simulink model "VehicleECU"  (R2018b)
settings: configuration reference "Active" (kept outside this file)
undefined symbols (not defined in the file): TUMHealthStatus, TUMStrategyState
settings Model: DataDictionary=VehicleECU.sldd  sg_rtwmakecfg_data=_sglibc_  ExplicitPartitioning=on  Creator=wischnewski  LastModifiedBy=ge34qer

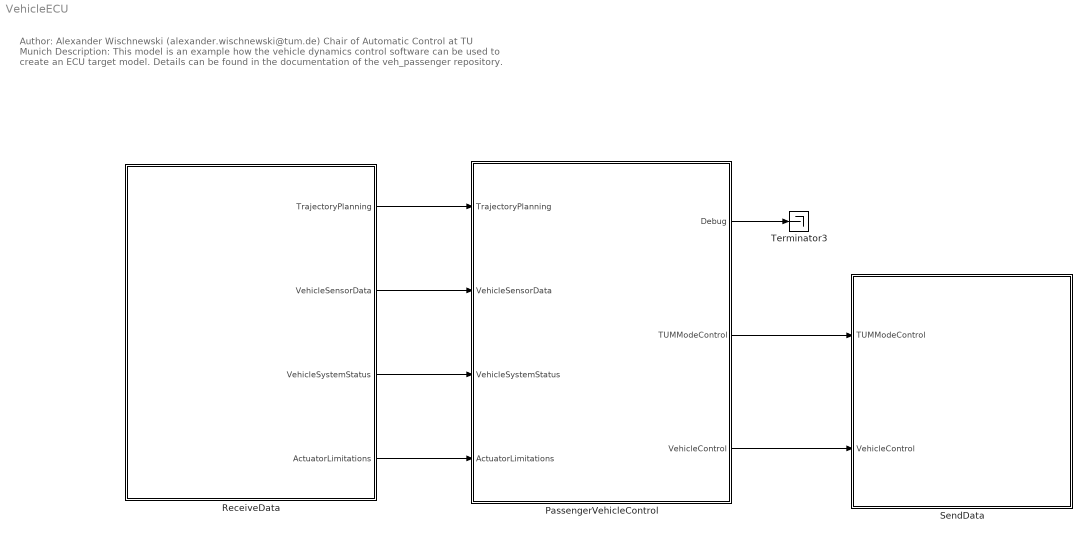
== system VehicleECU ==
  note: Author: Alexander Wischnewski (alexander.wischnewski@tum.de)
      | Chair of Automatic Control at TU Munich
      |
      | Description: This model is an example how the vehicle dynamics control software can be used to create an ECU target model. Details
      | can be found in the documentation of the veh_passenger repository.
  PassengerVehicleControl : Subsystem
  ReceiveData : Subsystem
  SendData : Subsystem
  Terminator3 : Terminator
  wires:
  ReceiveData/1(TrajectoryPlanning) -> PassengerVehicleControl/1(TrajectoryPlanning)
  ReceiveData/2(VehicleSensorData) -> PassengerVehicleControl/2(VehicleSensorData)
  ReceiveData/3(VehicleSystemStatus) -> PassengerVehicleControl/3(VehicleSystemStatus)
  ReceiveData/4(ActuatorLimitations) -> PassengerVehicleControl/4(ActuatorLimitations)
  PassengerVehicleControl/3(VehicleControl) -> SendData/2(VehicleControl)
  PassengerVehicleControl/2(TUMModeControl) -> SendData/1(TUMModeControl)
  PassengerVehicleControl/1(Debug) -> Terminator3/1

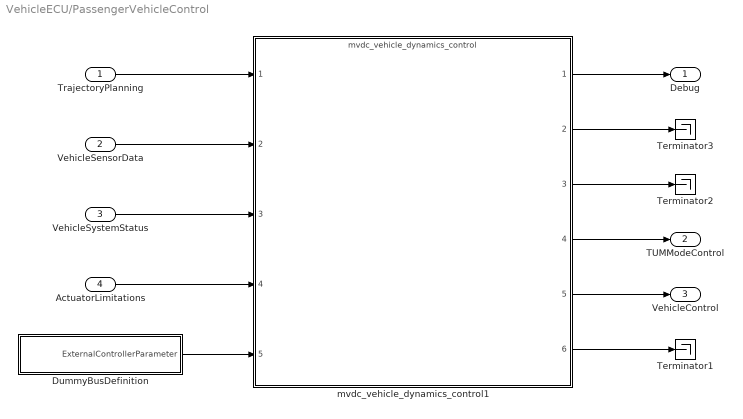
== system VehicleECU/PassengerVehicleControl ==
  TrajectoryPlanning : Inport
  VehicleSensorData : Inport  Port=2
  VehicleSystemStatus : Inport  Port=3
  ActuatorLimitations : Inport  Port=4
  DummyBusDefinition : Subsystem
  Terminator1 : Terminator
  Terminator2 : Terminator
  Terminator3 : Terminator
  mvdc_vehicle_dynamics_control1 : ModelReference  ModelNameDialog=mvdc_vehicle_dynamics_control  SimulationMode=Normal  ModelReferenceVersion=1.726
  Debug : Outport
  TUMModeControl : Outport  Port=2
  VehicleControl : Outport  Port=3
  wires:
  VehicleSystemStatus/1 -> mvdc_vehicle_dynamics_control1/3
  ActuatorLimitations/1 -> mvdc_vehicle_dynamics_control1/4
  VehicleSensorData/1 -> mvdc_vehicle_dynamics_control1/2
  TrajectoryPlanning/1 -> mvdc_vehicle_dynamics_control1/1
  mvdc_vehicle_dynamics_control1/6 -> Terminator1/1
  mvdc_vehicle_dynamics_control1/3 -> Terminator2/1
  mvdc_vehicle_dynamics_control1/2 -> Terminator3/1
  mvdc_vehicle_dynamics_control1/5 -> VehicleControl/1
  mvdc_vehicle_dynamics_control1/4 -> TUMModeControl/1
  DummyBusDefinition/1(ExternalControllerParameter) -> mvdc_vehicle_dynamics_control1/5
  mvdc_vehicle_dynamics_control1/1 -> Debug/1

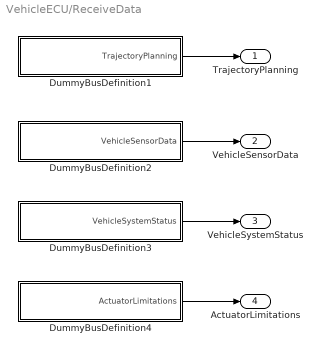
== system VehicleECU/ReceiveData ==
  DummyBusDefinition1 : Subsystem
  DummyBusDefinition2 : Subsystem
  DummyBusDefinition3 : Subsystem
  DummyBusDefinition4 : Subsystem
  TrajectoryPlanning : Outport
  VehicleSensorData : Outport  Port=2
  VehicleSystemStatus : Outport  Port=3
  ActuatorLimitations : Outport  Port=4
  wires:
  DummyBusDefinition4/1(ActuatorLimitations) -> ActuatorLimitations/1
  DummyBusDefinition3/1(VehicleSystemStatus) -> VehicleSystemStatus/1
  DummyBusDefinition2/1(VehicleSensorData) -> VehicleSensorData/1
  DummyBusDefinition1/1(TrajectoryPlanning) -> TrajectoryPlanning/1

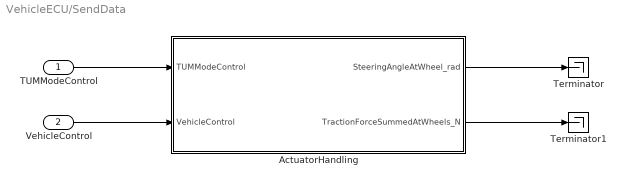
== system VehicleECU/SendData ==
  TUMModeControl : Inport  OutDataTypeStr=Bus: TUMModeControl
  VehicleControl : Inport  Port=2  OutDataTypeStr=Bus: VehicleControl
  ActuatorHandling : Subsystem
  Terminator : Terminator
  Terminator1 : Terminator
  wires:
  TUMModeControl/1 -> ActuatorHandling/1(TUMModeControl)
  VehicleControl/1 -> ActuatorHandling/2(VehicleControl)
  ActuatorHandling/1(SteeringAngleAtWheel_rad) -> Terminator/1
  ActuatorHandling/2(TractionForceSummedAtWheels_N) -> Terminator1/1

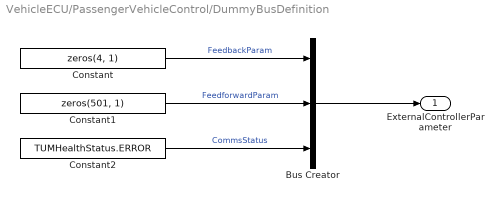
== system VehicleECU/PassengerVehicleControl/DummyBusDefinition ==
  Bus Creator : BusCreator  Inputs=3
  Constant : Constant  Value=zeros(4, 1)
  Constant1 : Constant  Value=zeros(501, 1)
  Constant2 : Constant  Value=TUMHealthStatus.ERROR
  ExternalControllerParameter : Outport
  wires:
  Bus Creator/1 -> ExternalControllerParameter/1
  Constant/1 -> Bus Creator/1  "FeedbackParam"
  Constant1/1 -> Bus Creator/2  "FeedforwardParam"
  Constant2/1 -> Bus Creator/3  "CommsStatus"

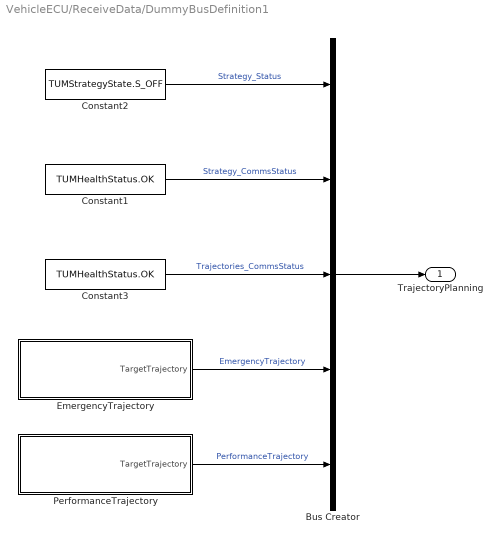
== system VehicleECU/ReceiveData/DummyBusDefinition1 ==
  Bus Creator : BusCreator  Inputs=5  OutDataTypeStr=Bus: TrajectoryPlanning
      settings: InheritFromInputs=off
  Constant1 : Constant  Value=TUMHealthStatus.OK
  Constant2 : Constant  Value=TUMStrategyState.S_OFF
  Constant3 : Constant  Value=TUMHealthStatus.OK
  EmergencyTrajectory : Subsystem  Priority=1000
  PerformanceTrajectory : Subsystem  Priority=1000
  TrajectoryPlanning : Outport
  wires:
  EmergencyTrajectory/1(TargetTrajectory) -> Bus Creator/4  "EmergencyTrajectory"
  Constant2/1 -> Bus Creator/1  "Strategy_Status"
  Constant1/1 -> Bus Creator/2  "Strategy_CommsStatus"
  Bus Creator/1 -> TrajectoryPlanning/1
  Constant3/1 -> Bus Creator/3  "Trajectories_CommsStatus"
  PerformanceTrajectory/1(TargetTrajectory) -> Bus Creator/5  "PerformanceTrajectory"

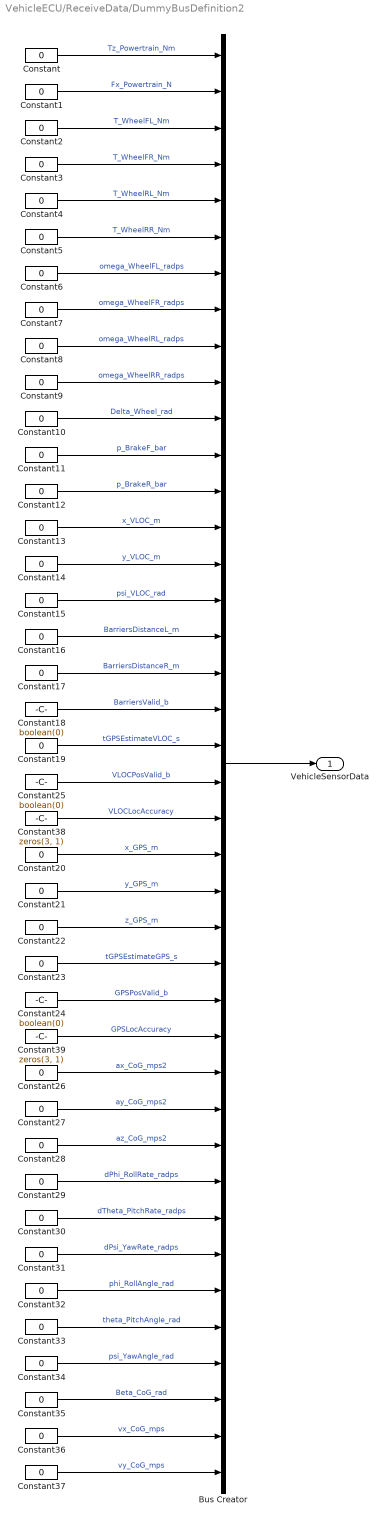
== system VehicleECU/ReceiveData/DummyBusDefinition2 ==
  Bus Creator : BusCreator  Inputs=40
  Constant{,1..17,19..23,26..37} (35 alike) : Constant  Value=0
  Constant18 : Constant  Value=boolean(0)
  Constant24 : Constant  Value=boolean(0)
  Constant25 : Constant  Value=boolean(0)
  Constant38 : Constant  Value=zeros(3, 1)
  Constant39 : Constant  Value=zeros(3, 1)
  VehicleSensorData : Outport
  wires:
  Bus Creator/1 -> VehicleSensorData/1
  Constant/1 -> Bus Creator/1  "Tz_Powertrain_Nm"
  Constant1/1 -> Bus Creator/2  "Fx_Powertrain_N"
  Constant2/1 -> Bus Creator/3  "T_WheelFL_Nm"
  Constant3/1 -> Bus Creator/4  "T_WheelFR_Nm"
  Constant4/1 -> Bus Creator/5  "T_WheelRL_Nm"
  Constant5/1 -> Bus Creator/6  "T_WheelRR_Nm"
  Constant6/1 -> Bus Creator/7  "omega_WheelFL_radps"
  Constant7/1 -> Bus Creator/8  "omega_WheelFR_radps"
  Constant8/1 -> Bus Creator/9  "omega_WheelRL_radps"
  Constant9/1 -> Bus Creator/10  "omega_WheelRR_radps"
  Constant10/1 -> Bus Creator/11  "Delta_Wheel_rad"
  Constant11/1 -> Bus Creator/12  "p_BrakeF_bar"
  Constant12/1 -> Bus Creator/13  "p_BrakeR_bar"
  Constant13/1 -> Bus Creator/14  "x_VLOC_m"
  Constant14/1 -> Bus Creator/15  "y_VLOC_m"
  Constant15/1 -> Bus Creator/16  "psi_VLOC_rad"
  Constant16/1 -> Bus Creator/17  "BarriersDistanceL_m"
  Constant17/1 -> Bus Creator/18  "BarriersDistanceR_m"
  Constant18/1 -> Bus Creator/19  "BarriersValid_b"
  Constant19/1 -> Bus Creator/20  "tGPSEstimateVLOC_s"
  Constant20/1 -> Bus Creator/23  "x_GPS_m"
  Constant21/1 -> Bus Creator/24  "y_GPS_m"
  Constant22/1 -> Bus Creator/25  "z_GPS_m"
  Constant23/1 -> Bus Creator/26  "tGPSEstimateGPS_s"
  Constant24/1 -> Bus Creator/27  "GPSPosValid_b"
  Constant25/1 -> Bus Creator/21  "VLOCPosValid_b"
  Constant26/1 -> Bus Creator/29  "ax_CoG_mps2"
  Constant27/1 -> Bus Creator/30  "ay_CoG_mps2"
  Constant28/1 -> Bus Creator/31  "az_CoG_mps2"
  Constant29/1 -> Bus Creator/32  "dPhi_RollRate_radps"
  Constant30/1 -> Bus Creator/33  "dTheta_PitchRate_radps"
  Constant31/1 -> Bus Creator/34  "dPsi_YawRate_radps"
  Constant32/1 -> Bus Creator/35  "phi_RollAngle_rad"
  Constant33/1 -> Bus Creator/36  "theta_PitchAngle_rad"
  Constant34/1 -> Bus Creator/37  "psi_YawAngle_rad"
  Constant35/1 -> Bus Creator/38  "Beta_CoG_rad"
  Constant36/1 -> Bus Creator/39  "vx_CoG_mps"
  Constant37/1 -> Bus Creator/40  "vy_CoG_mps"
  Constant38/1 -> Bus Creator/22  "VLOCLocAccuracy"
  Constant39/1 -> Bus Creator/28  "GPSLocAccuracy"

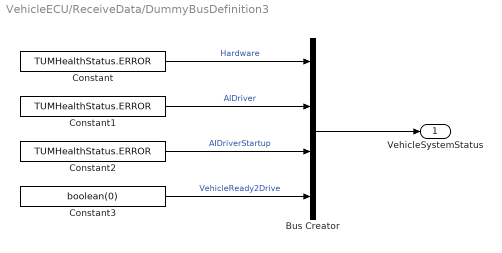
== system VehicleECU/ReceiveData/DummyBusDefinition3 ==
  Bus Creator : BusCreator  Inputs=4
  Constant : Constant  Value=TUMHealthStatus.ERROR
  Constant1 : Constant  Value=TUMHealthStatus.ERROR
  Constant2 : Constant  Value=TUMHealthStatus.ERROR
  Constant3 : Constant  Value=boolean(0)
  VehicleSystemStatus : Outport
  wires:
  Bus Creator/1 -> VehicleSystemStatus/1
  Constant/1 -> Bus Creator/1  "Hardware"
  Constant1/1 -> Bus Creator/2  "AIDriver"
  Constant2/1 -> Bus Creator/3  "AIDriverStartup"
  Constant3/1 -> Bus Creator/4  "VehicleReady2Drive"

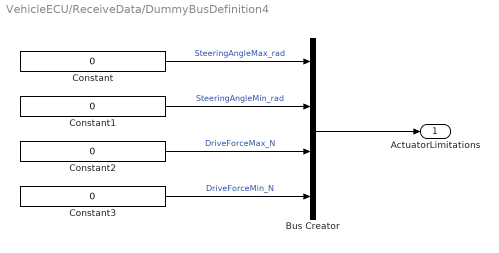
== system VehicleECU/ReceiveData/DummyBusDefinition4 ==
  Bus Creator : BusCreator  Inputs=4
  Constant{,1..3} (4 alike) : Constant  Value=0
  ActuatorLimitations : Outport
  wires:
  Bus Creator/1 -> ActuatorLimitations/1
  Constant/1 -> Bus Creator/1  "SteeringAngleMax_rad"
  Constant1/1 -> Bus Creator/2  "SteeringAngleMin_rad"
  Constant2/1 -> Bus Creator/3  "DriveForceMax_N"
  Constant3/1 -> Bus Creator/4  "DriveForceMin_N"

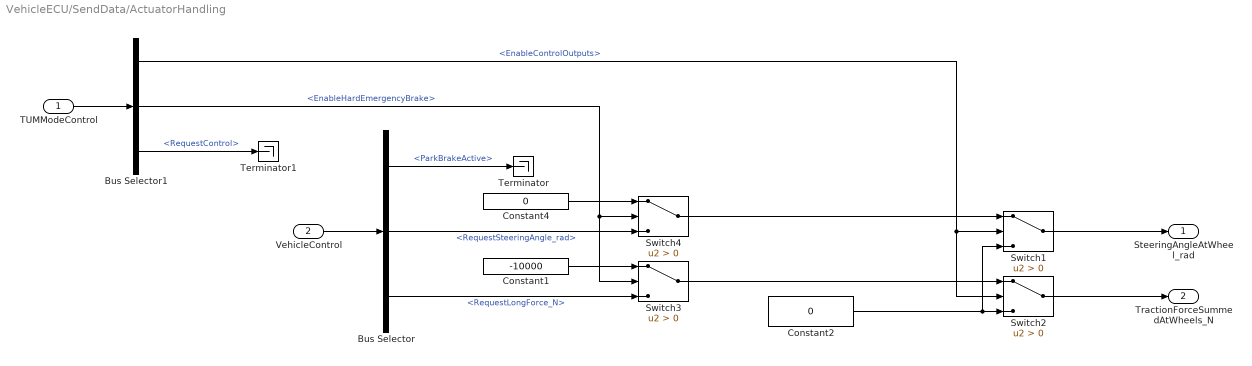
== system VehicleECU/SendData/ActuatorHandling ==
  TUMModeControl : Inport  OutDataTypeStr=Bus: TUMModeControl
  VehicleControl : Inport  Port=2  OutDataTypeStr=Bus: VehicleControl
  Bus Selector : BusSelector  OutputSignals=ParkBrakeActive,RequestSteeringAngle_rad,RequestLongForce_N
  Bus Selector1 : BusSelector  OutputSignals=EnableControlOutputs,EnableHardEmergencyBrake,RequestControl
  Constant1 : Constant  Value=-10000
  Constant2 : Constant  Value=0
  Constant4 : Constant  Value=0
  Switch{1..4} (4 alike) : Switch  Criteria=u2 > Threshold
  Terminator : Terminator
  Terminator1 : Terminator
  SteeringAngleAtWheel_rad : Outport
  TractionForceSummedAtWheels_N : Outport  Port=2
  wires:
  Bus Selector1/1 -> Switch2/2, Switch1/2  "<EnableControlOutputs>"
  TUMModeControl/1 -> Bus Selector1/1
  Bus Selector/3 -> Switch3/3  "<RequestLongForce_N>"
  Constant2/1 -> Switch1/3, Switch2/3
  VehicleControl/1 -> Bus Selector/1
  Bus Selector/2 -> Switch4/3  "<RequestSteeringAngle_rad>"
  Constant4/1 -> Switch4/1
  Constant1/1 -> Switch3/1
  Bus Selector1/2 -> Switch3/2, Switch4/2  "<EnableHardEmergencyBrake>"
  Bus Selector/1 -> Terminator/1  "<ParkBrakeActive>"
  Bus Selector1/3 -> Terminator1/1  "<RequestControl>"
  Switch4/1 -> Switch1/1
  Switch3/1 -> Switch2/1
  Switch1/1 -> SteeringAngleAtWheel_rad/1
  Switch2/1 -> TractionForceSummedAtWheels_N/1

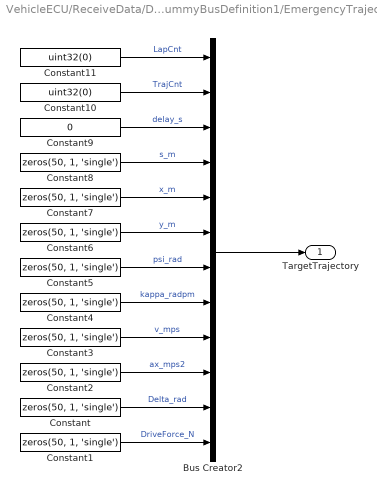
== system VehicleECU/ReceiveData/DummyBusDefinition1/EmergencyTrajectory ==
  Bus Creator2 : BusCreator  Inputs=12  OutDataTypeStr=Bus: Trajectory
      settings: InheritFromInputs=off
  Constant{,1..8} (9 alike) : Constant  Value=zeros(50, 1, 'single')
  Constant10 : Constant  Value=uint32(0)
  Constant11 : Constant  Value=uint32(0)
  Constant9 : Constant  Value=0
  TargetTrajectory : Outport  OutDataTypeStr=Bus: Trajectory
  wires:
  Constant8/1 -> Bus Creator2/4  "s_m"
  Constant7/1 -> Bus Creator2/5  "x_m"
  Constant6/1 -> Bus Creator2/6  "y_m"
  Constant5/1 -> Bus Creator2/7  "psi_rad"
  Constant4/1 -> Bus Creator2/8  "kappa_radpm"
  Constant3/1 -> Bus Creator2/9  "v_mps"
  Constant2/1 -> Bus Creator2/10  "ax_mps2"
  Constant11/1 -> Bus Creator2/1  "LapCnt"
  Constant10/1 -> Bus Creator2/2  "TrajCnt"
  Bus Creator2/1 -> TargetTrajectory/1
  Constant9/1 -> Bus Creator2/3  "delay_s"
  Constant/1 -> Bus Creator2/11  "Delta_rad"
  Constant1/1 -> Bus Creator2/12  "DriveForce_N"

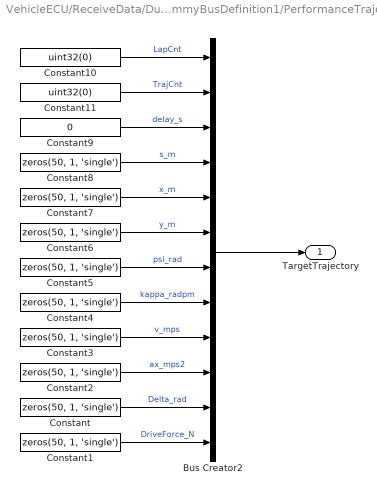
== system VehicleECU/ReceiveData/DummyBusDefinition1/PerformanceTrajectory ==
  Bus Creator2 : BusCreator  Inputs=12  OutDataTypeStr=Bus: Trajectory
      settings: InheritFromInputs=off
  Constant{,1..8} (9 alike) : Constant  Value=zeros(50, 1, 'single')
  Constant10 : Constant  Value=uint32(0)
  Constant11 : Constant  Value=uint32(0)
  Constant9 : Constant  Value=0
  TargetTrajectory : Outport  OutDataTypeStr=Bus: Trajectory
  wires:
  Constant8/1 -> Bus Creator2/4  "s_m"
  Constant7/1 -> Bus Creator2/5  "x_m"
  Constant6/1 -> Bus Creator2/6  "y_m"
  Constant5/1 -> Bus Creator2/7  "psi_rad"
  Constant4/1 -> Bus Creator2/8  "kappa_radpm"
  Constant3/1 -> Bus Creator2/9  "v_mps"
  Constant2/1 -> Bus Creator2/10  "ax_mps2"
  Constant10/1 -> Bus Creator2/1  "LapCnt"
  Constant11/1 -> Bus Creator2/2  "TrajCnt"
  Bus Creator2/1 -> TargetTrajectory/1
  Constant9/1 -> Bus Creator2/3  "delay_s"
  Constant/1 -> Bus Creator2/11  "Delta_rad"
  Constant1/1 -> Bus Creator2/12  "DriveForce_N"
